simulink model "Station_3_Handling_Sorting"  (R2024a)
settings: Solver=FixedStepAuto  StartTime=0.0  StopTime=30  FixedStep=0.05  RelTol=1e-3
libraries: opcualib x2
settings Model: Creator=admin  LastModifiedBy=admin

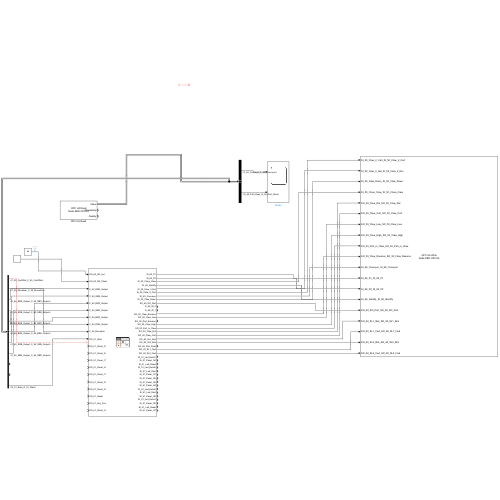
[thumbnail: Simulink's stored preview of the top-level diagram]
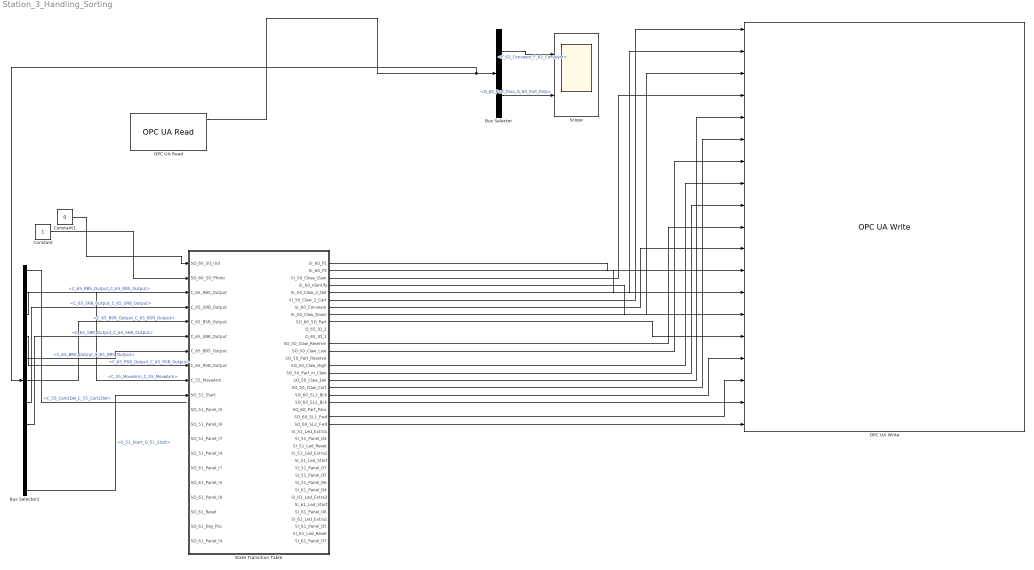
== system Station_3_Handling_Sorting ==
  Bus Selector : BusSelector  OutputSignals=F_62_Conveyor_F_62_Conveyor,O_60_Part_Pass_O_60_Part_Pass
  Bus Selector1 : BusSelector  OutputSignals=C_55_Cart2Del_C_55_Cart2Del,C_55_MoveArm_C_55_MoveArm,C_65_RBS_Output_C_65_RBS_Output,C_65_RSB_Output_C_65_RSB_Output,C_65_BRS_Output_C_65_BRS_Output,C_65_BSR_Output_C_65_BSR_Output,C_65_SRB_Output_C_65_SRB_Output,C_65_SBR_Output_C_65_SBR_Output,O_60_SInd_O_60_SInd,O_60_SPhoto_O_60_SPhoto,O_51_Start_O_51_Start
  Constant : Constant
  Constant1 : Constant  Value=0
  OPC UA Read : opcualib/OPC UA Read  SelectedServer=Node-RED OPCUA  ServerList=Node-RED OPCUA  NodeList={ '1', 'F_62_Conveyor', '15', 'F_62_Conveyor', '0'; '2', 'F_62_P1', '15', 'F_62_P1', '0'; '3', 'F_62_P2', '15', 'F_62_P2', '0'; '4', 'F_62_Identify', '15', 'F_62_Identify', '0'; '5', 'F_52_Claw_2_Del', '14', 'F_52_Claw_2_Del', '0'; '6', 'F_52_Claw_2_Cart', '14', 'F_52_Claw_2_Cart', '0'; '7', 'F_52_Claw_Down', '14', 'F_52_Claw_Down', '0'; '8', 'F_52_Close_Claw', '14', 'F_52_Close_Claw', '0'; '9', 'C_55_Cart2Del', '14', 'C_55_Cart2Del', '0'; '10', 'C_55_Del2Cart', '14', 'C_55_Del2Cart', '0'; '11', 'C_55_MoveArm', '14', 'C_55_MoveArm', '0'; '12', 'C_65_RBS_Output', '15', 'C_65_RBS_Output', '0'; '13', 'C_65_RSB_Output', '15', 'C_65_RSB_Output', '0'; '14', 'C_65_BRS_Output', '15', 'C_65_BRS_Output', '0'; '15', 'C_65_BSR_Output', '15', 'C_65_BSR_Output', '0'; '16', 'C_65_SRB_Output', '15', 'C_65_SRB_Output', '0'; '17', 'C_65_SBR_Output', '15', 'C_65_SBR_Output', '0'; '18', 'O_60_SInd', '15', 'O_60_SInd', '0'; '19', 'O_60_SPhoto', '15', 'O_60_SPhoto', '0'; '20', 'O_50_Claw_Cart', '14', 'O_50_Claw_Cart', '0'; '21', 'O_50_Claw_Del', '14', 'O_50_Claw_Del', '0'; '22', 'O_50_Claw_Low', '14', 'O_50_Claw_Low', '0'; '23', 'O_50_Claw_High', '14', 'O_50_Claw_High', '0'; '24', 'O_50_Part_in_Claw', '14', 'O_50_Part_in_Claw', '0'; '25', 'O_60_Part_Pass', '15', 'O_60_Part_Pass', '0'; '26', 'O_60_SL2_Bck', '15', 'O_60_SL2_Bck', '0'; '27', 'O_60_SL2_Fwd', '15', 'O_60_SL2_Fwd', '0'; '28', 'O_60_SPart', '15', 'O_60_SPart', '0'; '29', 'O_51_Start', '14', 'O_51_Start', '0'; '30', 'O_60_SL1_Bck', '15', 'O_60_SL1_Bck', '0'; '31', 'O_60_SL1_Fwd', '15', 'O_60_SL1_Fwd', '0' }  ShowQualityPort=on  ShowTimestampPort=on  ShowTimestampPortAs=Seconds since start  SampleTime=-1
  OPC UA Write : opcualib/OPC UA Write  SelectedServer=Node-RED OPCUA  ServerList=Node-RED OPCUA  SampleTime=-1  NodeList={ '1', 'SI_50_Claw_2_Cart', '14', 'SI_50_Claw_2_Cart', '0'; '2', 'SI_50_Claw_2_Del', '14', 'SI_50_Claw_2_Del', '0'; '3', 'SI_50_Claw_Down', '14', 'SI_50_Claw_Down', '0'; '4', 'SI_50_Close_Claw', '14', 'SI_50_Close_Claw', '0'; '5', 'SO_50_Claw_Del', '14', 'SO_50_Claw_Del', '0'; '6', 'SO_50_Claw_Cart', '14', 'SO_50_Claw_Cart', '0'; '7', 'SO_50_Claw_Low', '14', 'SO_50_Claw_Low', '0'; '8', 'SO_50_Claw_High', '14', 'SO_50_Claw_High', '0'; '9', 'SO_50_Part_in_Claw', '14', 'SO_50_Part_in_Claw', '0'; '10', 'SO_50_Claw_Reserve', '14', 'SO_50_Claw_Reserve', '0'; '11', 'SI_60_Conveyor', '15', 'SI_60_Conveyor', '0'; '12', 'SI_60_P1', '15', 'SI_60_P1', '0'; '13', 'SI_60_P2', '15', 'SI_60_P2', '0'; '14', 'SI_60_Identify', '15', 'SI_60_Identify', '0'; '15', 'SO_60_SO_Part', '15', 'SO_60_SO_Part', '0'; '16', 'SO_60_SL1_Bck', '15', 'SO_60_SL1_Bck', '0'; '17', 'SO_60_SL1_Fwd', '15', 'SO_60_SL1_Fwd', '0'; '18', 'SO_60_SL2_Bck', '15', 'SO_60_SL2_Bck', '0'; '19', 'SO_60_SL2_Fwd', '15', 'SO_60_SL2_Fwd', '0' }
  Scope : Scope  NumInputPorts=2
  State Transition Table : State Transition Table  TreatAsAtomicUnit=on
  wires:
  OPC UA Read/1 -> Bus Selector1/1, Bus Selector/1
  Bus Selector1/1 -> ?  "<C_55_Cart2Del_C_55_Cart2Del>"
  Bus Selector1/2 -> State Transition Table/9(C_55_MoveArm)  "<C_55_MoveArm_C_55_MoveArm>"
  Bus Selector1/3 -> State Transition Table/3(C_65_RBS_Output)  "<C_65_RBS_Output_C_65_RBS_Output>"
  Bus Selector1/4 -> State Transition Table/8(C_65_RSB_Output)  "<C_65_RSB_Output_C_65_RSB_Output>"
  Bus Selector1/5 -> State Transition Table/7(C_65_BRS_Output)  "<C_65_BRS_Output_C_65_BRS_Output>"
  Bus Selector1/6 -> State Transition Table/5(C_65_BSR_Output)  "<C_65_BSR_Output_C_65_BSR_Output>"
  Bus Selector1/7 -> State Transition Table/4(C_65_SRB_Output)  "<C_65_SRB_Output_C_65_SRB_Output>"
  Bus Selector1/8 -> State Transition Table/6(C_65_SBR_Output)  "<C_65_SBR_Output_C_65_SBR_Output>"
  ? -> ?
  Constant1/1 -> State Transition Table/1(SO_60_SO_Ind)
  Bus Selector1/11 -> State Transition Table/10(SO_51_Start)  "<O_51_Start_O_51_Start>"
  Bus Selector/1 -> Scope/1  "<F_62_Conveyor_F_62_Conveyor>"
  Bus Selector/2 -> Scope/2  "<O_60_Part_Pass_O_60_Part_Pass>"
  State Transition Table/1(SI_60_P1) -> OPC UA Write/12
  State Transition Table/2(SI_60_P2) -> OPC UA Write/13
  State Transition Table/6(SI_50_Claw_2_Cart) -> OPC UA Write/1
  State Transition Table/5(SI_50_Claw_2_Del) -> OPC UA Write/2
  State Transition Table/8(SI_50_Claw_Down) -> OPC UA Write/3
  State Transition Table/3(SI_50_Close_Claw) -> OPC UA Write/4
  State Transition Table/17(SO_50_Claw_Del) -> OPC UA Write/5
  State Transition Table/18(SO_50_Claw_Cart) -> OPC UA Write/6
  State Transition Table/13(SO_50_Claw_Low) -> OPC UA Write/7
  State Transition Table/15(SO_50_Claw_High) -> OPC UA Write/8
  State Transition Table/16(SO_50_Part_in_Claw) -> OPC UA Write/9
  State Transition Table/12(SO_50_Claw_Reserve) -> OPC UA Write/10
  State Transition Table/7(SI_60_Conveyor) -> OPC UA Write/11
  State Transition Table/4(SI_60_Identify) -> OPC UA Write/14
  State Transition Table/9(SO_60_SO_Part) -> OPC UA Write/15
  State Transition Table/19(SO_60_SL1_Bck) -> OPC UA Write/16
  State Transition Table/22(SO_60_SL1_Fwd) -> OPC UA Write/17
  State Transition Table/20(SO_60_SL2_Bck) -> OPC UA Write/18
  State Transition Table/23(SO_60_SL2_Fwd) -> OPC UA Write/19
  Constant/1 -> State Transition Table/2(SO_60_SO_Photo)

== stateflow chart Station_3_Handling_Sorting/State Transition Table ==
  state state1
    SI_50_Claw_2_Cart=0;
    SI_50_Claw_2_Del=0;
    SI_50_Claw_Down=0;
    SI_50_Close_Claw=0;
    SI_60_Conveyor=0;
    SI_60_P1=0;
    SI_60_P2=0;
    SI_60_Identify=0;
    SO_60_SO_Part=0;
    SO_60_SO_Ind;
    SO_60_SO_Photo;
    C_65_RBS_Output;
    C_65_RSB_Output;
    C_65_BRS_Output;
    C_65_BSR_Output;
    C_65_SRB_Output;
    C_65_SBR_Output;
    SO_50_Part_Reserve=0;
    SO_50_Claw_Del=0;
    SO_50_Claw_Reserve=0;
    SO_50_Claw_Cart=1;
    SO_50_Claw_Low=0;
    SO_50_Claw_High=1;
    SO_50_Part_in_Claw=0;
    SO_60_SO_Part=0;
    SO_60_Part_Pass=0;
    SO_60_SL1_Bck=1;
    SO_60_SL1_Fwd=0;
    SO_60_SL2_Bck=1;
    SO_60_SL2_Fwd=0;
    SO_51_Panel_I4;
    SO_51_Panel_I5;
    SO_51_Panel_I6;
    SO_51_Panel_I7;
    SI_51_Led_Start;
    SI_51_Led_Reset;
    SI_51_Led_Extra1=0;
    SI_51_Led_Extra2=0;
    SI_51_Panel_O4;
    SI_51_Panel_O5;
    SI_51_Panel_O6;
    SI_51_Panel_O7;
    SO_61_Key_Pos;
    SO_61_Reset;
    SO_61_Panel_I4;
    SO_61_Panel_I5;
    SO_61_Panel_I6;
    SO_61_Panel_I7;
    SI_61_Led_Start=0;
    SI_61_Led_Reset;
    SI_61_Led_Extra1=0;
    SI_61_Led_Extra2=0;
    SI_61_Panel_O4;
    SI_61_Panel_O5;
    SI_61_Panel_O6;
    SI_61_Panel_O7;
  state state2
  state CLAW_DOWN
    SI_50_Claw_2_Cart=0;
    SI_50_Claw_2_Del=0;
    SI_50_Claw_Down=1;
    SI_50_Close_Claw=0;
    state CLAW_DOWN_1
    (default) -> CLAW_DOWN_1
    CLAW_DOWN_1 -> (junction 215) : after(0.2,sec)
        | {SO_50_Claw_High=0;}
    (junction 215) -> CLAW_DOWN_1
  state CLAW_UP
    SI_50_Claw_2_Cart=0;
    SI_50_Claw_2_Del=0;
    SI_50_Claw_Down=0;
    SI_50_Close_Claw=1;
    state CLAW_UP_1
    (default) -> CLAW_UP_1
    CLAW_UP_1 -> (junction 219) : after(0.2,sec)
        | {SO_50_Claw_Low=0;}
    (junction 219) -> CLAW_UP_1
  state CLAW_TO_DEL
    SI_50_Claw_2_Cart=0;
    SI_50_Claw_2_Del=1;
    SI_50_Claw_Down=0;
    SI_50_Close_Claw=1;
    state CLAW_TO_DEL_1
    state CLAW_TO_DEL_2
    state CLAW_TO_DEL_3
    CLAW_TO_DEL_3 -> (junction 188) : after(0.05,sec)
        | {SO_50_Claw_Reserve=0;}
    (default) -> CLAW_TO_DEL_1
    CLAW_TO_DEL_1 -> CLAW_TO_DEL_2 : after(0.25,sec)
        | {SO_50_Claw_Cart=0;}
    CLAW_TO_DEL_2 -> CLAW_TO_DEL_3 : after(0.5,sec)
        | {SO_50_Claw_Reserve=1;}
    (junction 188) -> CLAW_TO_DEL_3
  state CLAW_DOWN_DEL
    SI_50_Claw_2_Cart=0;
    SI_50_Claw_2_Del=0;
    SI_50_Claw_Down=1;
    SI_50_Close_Claw=1;
    state CLAW_DOWN_DEL_1
    (default) -> CLAW_DOWN_DEL_1
    CLAW_DOWN_DEL_1 -> (junction 389) : after(0.2,sec)
        | {SO_50_Claw_High=0;}
    (junction 389) -> CLAW_DOWN_DEL_1
  state back_to_cart
    SI_60_Conveyor=1;
    SI_60_P1=0;
    SI_60_P2=0;
    SI_60_Identify=0;
    SI_50_Close_Claw=0;
    state back_to_cart_1
    state back_to_cart_2
    state back_to_cart_4
    state back_to_cart_3
    back_to_cart_3 -> (junction 394) : after(0.35,sec)
        | {SO_50_Claw_Del=0;}
    (default) -> back_to_cart_1
    back_to_cart_1 -> back_to_cart_2 : after(0.2,sec)
        | {SO_50_Claw_Low=0;}
    back_to_cart_2 -> back_to_cart_4 : after(0.3,sec)
        | {SO_60_SO_Part=0;}
    back_to_cart_4 -> back_to_cart_3 : after(0.45,sec)
        | {SI_50_Claw_2_Cart=1;
        | SO_50_Claw_High=1;}
    (junction 394) -> back_to_cart_3
  state decision
  state P1
    SI_60_Conveyor=1;
    SI_60_P1=1;
    SI_60_P2=0;
    state P1_1
      state P1_1_1
      (default) -> P1_1_1
      P1_1_1 -> (junction 291) : after(0.2,sec)
          | {SO_60_SL1_Bck=0;}
      (junction 291) -> P1_1_1
    state P1_2
      state P1_2_1
      state P1_2_2
      P1_2_2 -> (junction 178) : after(0.05,sec)
          | {SO_50_Claw_Reserve=0;}
      (default) -> P1_2_1
      P1_2_1 -> P1_2_2 : after(0.1,sec)
          | {SO_50_Claw_Reserve=1;}
      (junction 178) -> P1_2_2
    (junction 225) -> P1_2
    (default) -> P1_1
    P1_1 -> P1_2 : after(0.4,sec)
        | {SI_60_Identify=1;
        | SO_60_SL1_Fwd=1;}
    P1_2 -> (junction 225) : after(0.55,sec)
        | {SI_50_Claw_2_Cart=0;
        | SO_50_Claw_Cart=1;}
  state P1_END
    SI_60_Conveyor=0;
    SI_60_P1=0;
    SI_60_P2=0;
    state P1_END_1
      state P1_END_1_1
      (default) -> P1_END_1_1
      P1_END_1_1 -> (junction 258) : after(0.15,sec)
          | {SO_60_SL1_Fwd=0;}
      (junction 258) -> P1_END_1_1
    (default) -> P1_END_1
    P1_END_1 -> (junction 254) : after(0.2,sec)
        | {SO_60_Part_Pass=0;}
    (junction 254) -> P1_END_1
  state P2
    SI_60_Conveyor=1;
    SI_60_P1=0;
    SI_60_P2=1;
    state P2_1
      state P2_1_1
      (default) -> P2_1_1
      P2_1_1 -> (junction 295) : after(0.2,sec)
          | {SO_60_SL2_Bck=0;}
      (junction 295) -> P2_1_1
    state P2_2
      state P2_2_1
      state P2_2_2
      P2_2_2 -> (junction 204) : after(0.05,sec)
          | {SO_50_Claw_Reserve=0;}
      (default) -> P2_2_1
      P2_2_1 -> P2_2_2 : after(0.1,sec)
          | {SO_50_Claw_Reserve=1;}
      (junction 204) -> P2_2_2
    (junction 141) -> P2_2
    (default) -> P2_1
    P2_1 -> P2_2 : after(0.4,sec)
        | {SI_60_Identify=1;
        | SO_60_SL2_Fwd=1;}
    P2_2 -> (junction 141) : after(0.55,sec)
        | {SI_50_Claw_2_Cart=0;
        | SO_50_Claw_Cart=1;}
  state P2_END
    state P2_END_1
      state P2_END_1_1
      (default) -> P2_END_1_1
      P2_END_1_1 -> (junction 273) : after(0.15,sec)
          | {SO_60_SL2_Fwd=0;}
      (junction 273) -> P2_END_1_1
    (default) -> P2_END_1
    P2_END_1 -> (junction 277) : after(0.2,sec)
        | {SO_60_Part_Pass=0;}
    (junction 277) -> P2_END_1
  state none
    SI_60_Conveyor=1;
    SI_60_Identify=1;
    SI_60_P1=0;
    SI_60_P2=0;
    state none_1
    state none_2
    state none_3
    none_3 -> (junction 316) : after(0.25,sec)
        | {SI_50_Claw_2_Cart=0;
        | SO_50_Claw_Cart=1;}
    (default) -> none_1
    none_1 -> none_2 : after(0.65,sec)
        | {SO_50_Claw_Reserve=1;}
    none_2 -> none_3 : after(0.05,sec)
        | {SO_50_Claw_Reserve=0;}
    (junction 316) -> none_3
  state NONE_END
    SI_60_Conveyor=0;
    SI_60_Identify=0;
    SI_60_P1=0;
    SI_60_P2=0;
  (default) -> state1
  (junction 53) -> state1
  (junction 284) -> (junction 53)
  state1 -> state2 : [(SO_51_Start==1 ||  C_55_MoveArm==1)]
  state2 -> CLAW_DOWN : after(0.15,sec)
  CLAW_DOWN -> CLAW_UP : after(0.7,sec)
      | {SO_50_Claw_Low=1;
      | SO_50_Part_in_Claw=1;}
  CLAW_UP -> CLAW_TO_DEL : after(0.95,sec)
      | {SO_50_Claw_High=1;}
  CLAW_TO_DEL -> CLAW_DOWN_DEL : after(2.3,sec)
      | {SO_50_Claw_Del=1;}
  CLAW_DOWN_DEL -> back_to_cart : after(0.7,sec)
      | {SI_50_Claw_Down=0;
      | SO_50_Claw_Low=1;
      | SO_50_Part_in_Claw=0;
      | SO_60_SO_Part=1;}
  back_to_cart -> decision [order 1] : [SO_60_SO_Ind==1 &&after(2,sec)]
      | {O_65_ID_1=0;
      | O_65_ID_2=1;}
  back_to_cart -> decision [order 2] : [(SO_60_SO_Ind==0 && SO_60_SO_Photo==1) &&after(2,sec)]
      | {O_65_ID_1=1;
      | O_65_ID_2=1;
      | }
  back_to_cart -> decision [order 3] : [(SO_60_SO_Ind==0 && SO_60_SO_Photo==0)&&after(2,sec)]
      | {O_65_ID_1=1;
      | O_65_ID_2=0;}
  decision -> (junction 369) [order 2] : [((((O_65_ID_1==1&&O_65_ID_2==1)&&( C_65_BRS_Output==1 || C_65_SRB_Output==1)))||(((O_65_ID_1==1&&O_65_ID_2==0)&&( C_65_SBR_Output==1 || C_65_RBS_Output==1)))||(((O_65_ID_1==0 && O_65_ID_2==1)&&( C_65_RSB_Output==1 || C_65_BSR_Output==1))))]
  (junction 369) -> (junction 64)
  decision -> (junction 372) [order 3] : [((((O_65_ID_1==1&&O_65_ID_2==1)&&( C_65_BSR_Output==1 || C_65_SBR_Output==1)))||(((O_65_ID_1==1&&O_65_ID_2==0)&&( C_65_SRB_Output==1 || C_65_RSB_Output==1)))||(((O_65_ID_1==0 && O_65_ID_2==1)&&( C_65_RBS_Output==1 || C_65_BRS_Output==1))))]
  (junction 372) -> (junction 81)
  decision -> P1 [order 1] : [((((O_65_ID_1==1&&O_65_ID_2==1)&&( C_65_RBS_Output==1  || C_65_RSB_Output==1)))||(((O_65_ID_1==1&&O_65_ID_2==0)&&( C_65_BRS_Output==1 ||  C_65_BSR_Output==1)))||(((O_65_ID_1==0 && O_65_ID_2==1)&&( C_65_SRB_Output==1 || C_65_SBR_Output==1))))]
  P1 -> P1_END : after(2.4,sec)
      | {SI_60_Identify=0;
      | SO_60_Part_Pass=1;}
  P1_END -> (junction 284) : after(0.3,sec)
      | {SO_60_SL1_Bck=1;}
  (junction 281) -> (junction 284)
  (junction 64) -> P2
  P2 -> P2_END : after(3,sec)
      | {SI_60_Identify=0;
      | SO_60_Part_Pass=1;}
  P2_END -> (junction 281) : after(0.3,sec)
      | {SO_60_SL2_Bck=1;}
  (junction 288) -> (junction 281)
  (junction 81) -> none
  none -> NONE_END : after(3,sec)
      | {SO_60_Part_Pass=1;}
  NONE_END -> (junction 288) : after(0.2,sec)
      | {SO_60_Part_Pass=0;}
  data: SI_60_P1 output; SI_60_P2 output; SI_50_Close_Claw output; SI_60_Identify output; SI_50_Claw_2_Del output; SI_50_Claw_2_Cart output; SI_60_Conveyor output; SI_50_Claw_Down output; SO_60_SO_Ind input; SO_60_SO_Photo input; SO_60_SO_Part output; O_65_ID_2 output; O_65_ID_1 output; C_65_RBS_Output input; C_65_SRB_Output input; C_65_BSR_Output input; C_65_SBR_Output input; C_65_BRS_Output input; C_65_RSB_Output input; SO_50_Claw_Reserve output; SO_50_Claw_Low output; SO_50_Part_Reserve output; SO_50_Claw_High output; SO_50_Part_in_Claw output; SO_50_Claw_Del output; SO_50_Claw_Cart output; SO_60_SL1_Bck output; SO_60_SL2_Bck output; SO_60_Part_Pass output; SO_60_SL1_Fwd output; SO_60_SL2_Fwd output; C_55_MoveArm input; SO_51_Start input; SO_51_Panel_I5 input; SO_51_Panel_I6 input; SO_51_Panel_I7 input; SO_51_Panel_I4 input; SI_51_Led_Extra1 output; SI_51_Panel_O4 output =0; SI_51_Led_Reset output =0; SI_51_Led_Extra2 output; SI_51_Led_Start output =0; SI_51_Panel_O7 output =0; SI_51_Panel_O5 output =0; SI_51_Panel_O6 output =0; SO_61_Panel_I7 input; SO_61_Panel_I5 input; SO_61_Panel_I6 input; SO_61_Reset input; SO_61_Key_Pos input; SO_61_Panel_I4 input; SI_61_Panel_O4 output =0; SI_61_Led_Extra2 output; SI_61_Led_Start output; SI_61_Panel_O6 output =0; SI_61_Led_Extra1 output; SI_61_Panel_O5 output =0; SI_61_Led_Reset output =0; SI_61_Panel_O7 output =0
